simulink model "mSimpleLongWhl"  (R2019b)
settings: Solver=ode4  StartTime=0.0  StopTime=30  FixedStep=0.001  RelTol=1e-3
model workspace (MAT data in the model file):
  C_rr = 0.05
  MaxBrkPrs = 80000
  MaxBrkTrq = 500
  TireLoadedRadius = 0.5
  WhlFz = 3000
  w_thresh = 0.1
libraries: VsrLibWheel x1
settings Model: Creator=9bt  LastModifiedBy=4qz

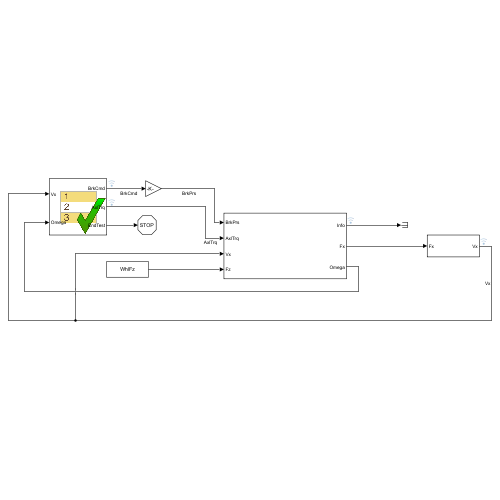
[thumbnail: Simulink's stored preview of the top-level diagram]
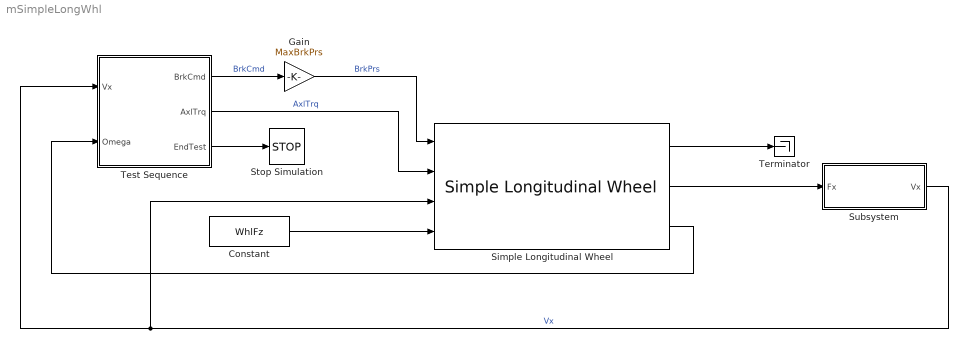
== system mSimpleLongWhl ==
  Constant : Constant  Value=WhlFz
  Gain : Gain  Gain=MaxBrkPrs
  Simple Longitudinal Wheel : VsrLibWheel/Simple Longitudinal Wheel  TireLoadedRadius=TireLoadedRadius  C_rr=C_rr  MaxBrkTrq=MaxBrkTrq  MaxBrkPrs=MaxBrkPrs  w_thresh=w_thresh
  Stop Simulation : Stop
  Subsystem : Subsystem
  Terminator : Terminator
  Test Sequence : Test Sequence  TreatAsAtomicUnit=on
  wires:
  Simple Longitudinal Wheel/2 -> Subsystem/1(Fx)
  Constant/1 -> Simple Longitudinal Wheel/4
  Subsystem/1(Vx) -> Simple Longitudinal Wheel/3, Test Sequence/1(Vx)  "Vx"
  Test Sequence/1(BrkCmd) -> Gain/1  "BrkCmd"
  Test Sequence/2(AxlTrq) -> Simple Longitudinal Wheel/2  "AxlTrq"
  Simple Longitudinal Wheel/1 -> Terminator/1
  Simple Longitudinal Wheel/3 -> Test Sequence/2(Omega)
  Test Sequence/3(EndTest) -> Stop Simulation/1
  Gain/1 -> Simple Longitudinal Wheel/1  "BrkPrs"

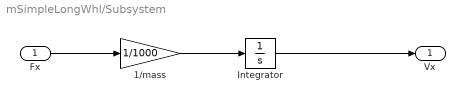
== system mSimpleLongWhl/Subsystem ==
  Fx : Inport
  1/mass : Gain  Gain=1/1000
  Integrator : Integrator
  Vx : Outport
  wires:
  Fx/1 -> 1/mass/1
  Integrator/1 -> Vx/1
  1/mass/1 -> Integrator/1

== stateflow chart mSimpleLongWhl/Test Sequence ==
  settings: stateMachineType=SIMPLIFIED_MACHINE
  state Init
    BrkCmd = 0;
    AxlTrq = 0;
    EndTest = false;
  state CheckBrkStopped
    BrkCmd = 1;
    state NoAxlTrq
      BrkCmd = 1;
      AxlTrq = 0;
      verify(abs(Omega) <= 1e-6)
    state PosAxlTrq
      BrkCmd = 1;
      AxlTrq = 200;
      verify(Omega <= w_thresh)
    state NegAxlTrq
      BrkCmd = 1;
      AxlTrq = -200;
      verify(abs(Omega) <= w_thresh)
    (default) -> NoAxlTrq
    NoAxlTrq -> PosAxlTrq : [
        | after(1,sec)
        | ]
    PosAxlTrq -> NegAxlTrq : [
        | after(1,sec)
        | ]
  state Acceleration
    BrkCmd = 0;
    AxlTrq = 500;
    state WaitForPositiveSpd
    state CheckPositiveSpd
      verify(Vx > 0 && Omega > 0)
    (default) -> WaitForPositiveSpd
    WaitForPositiveSpd -> CheckPositiveSpd : [
        | after(.1,sec)
        | ]
  state Braking
    BrkCmd = .9;
    AxlTrq = 0;
    verify(Vx > 0 && Omega > 0)
  state EndTest
    EndTest = true;
  (default) -> Init
  Init -> CheckBrkStopped : [
      | true
      | ]
  CheckBrkStopped -> Acceleration : [
      | after(3,sec)
      | ]
  Acceleration -> Braking [order 1] : [
      | Vx > 5
      | ]
  Acceleration -> Braking [order 2] : [
      | after(10, sec)
      | ]
  Braking -> EndTest : [
      | after(10, sec)
      | ]
  data: BrkCmd output size=1; AxlTrq output; Vx input; Omega input; w_thresh parameter; EndTest output
